simulink model "tank_PI"  (R2021a)
settings: Solver=FixedStepAuto  StartTime=0.0  StopTime=inf  FixedStep=0.1  RelTol=1e-3
model workspace (MATLAB code in the model file):
  | A1 = 1;
  | a1 = 0.1*0.1;
  | A2 = A1;
  | a2 = a1;
  | h10 = 1;
  | h20=1;
settings Model: EnablePacing=on  PacingRate=10  Creator=kjartan  LastModifiedBy=kjartan
settings SolverCC: AlgebraicLoopSolver=TrustRegion
settings DataIOCC: ReturnWorkspaceOutputs=off
settings DebuggingCC: SFMachineParentedDataDiag=warning  ArithmeticOperatorsInVariantConditions=warning
settings SFSimCC: CustomCodeUndefinedFunction=UseInterfaceOnly

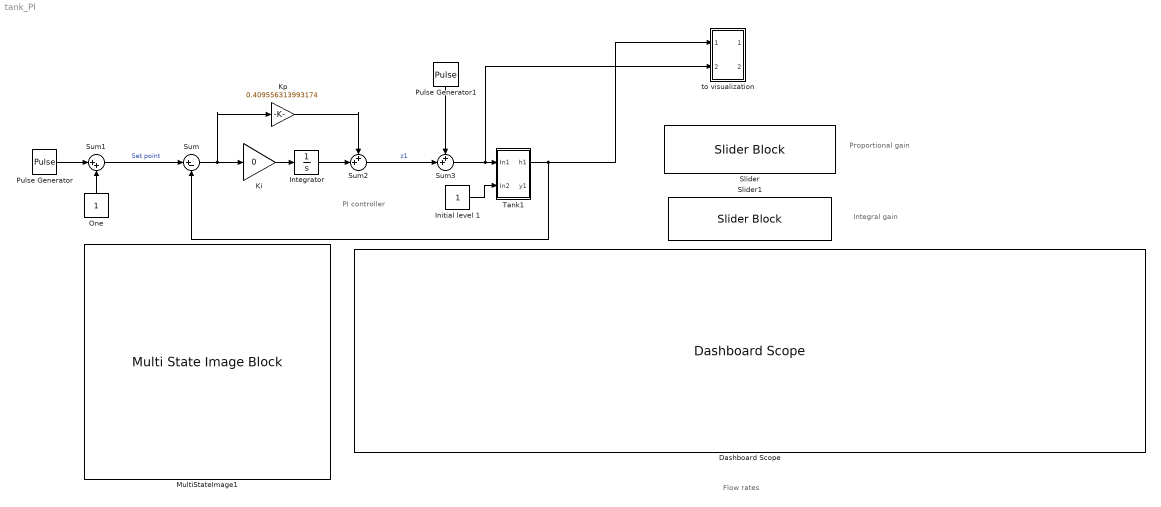
== system tank_PI ==
  note: Proportional gain
  note: Flow rates
  note: PI controller
  note: Integral gain
  Dashboard Scope : DashboardScope  Ymin=0  Ymax=2.5  ScaleAtStop=off
  Initial level 1 : Constant
  Integrator : Integrator
  Ki : Gain  Gain=0
  Kp : Gain  Gain=0.409556313993174
  MultiStateImage1 : MultiStateImageBlock
  One : Constant  OutDataTypeStr=Inherit: Inherit via back propagation
  Pulse Generator : DiscretePulseGenerator  PulseType=Time based  Amplitude=0.5  Period=60  PulseWidth=50
  Pulse Generator1 : DiscretePulseGenerator  PulseType=Time based  Amplitude=0.1  Period=60  PulseWidth=25  PhaseDelay=15
  Slider : SliderBlock  ScaleMax=2
  Slider1 : SliderBlock  ScaleMax=2
  Sum : Sum  Inputs=|+-
  Sum1 : Sum  Inputs=|++
  Sum2 : Sum  Inputs=++|
  Sum3 : Sum  Inputs=++|
  Tank1 : Subsystem
  to visualization : Subsystem
  wires:
  Tank1/1(h1) -> to visualization/1(In2), Sum/2
  Pulse Generator/1 -> Sum1/1
  Integrator/1 -> Sum2/2
  Sum/1 -> Kp/1, Ki/1
  Ki/1 -> Integrator/1
  Sum2/1 -> Sum3/2  "z1"
  Initial level 1/1 -> Tank1/2(In2)
  Kp/1 -> Sum2/1
  One/1 -> Sum1/2
  Sum1/1 -> Sum/1  "Set point"
  Sum3/1 -> to visualization/2(In3), Tank1/1(In1)
  Pulse Generator1/1 -> Sum3/1

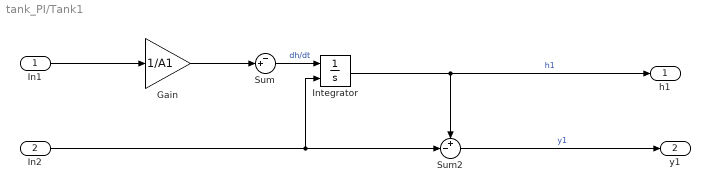
== system tank_PI/Tank1 ==
  In1 : Inport
  In2 : Inport  Port=2
  Gain : Gain  Gain=1/A1
  Integrator : Integrator  InitialConditionSource=external  InitialCondition=h10  LimitOutput=on  LowerSaturationLimit=0
  Sum : Sum  Inputs=-+|
  Sum2 : Sum  Inputs=+-|
  h1 : Outport  VectorParamsAs1DForOutWhenUnconnected=off
  y1 : Outport  Port=2  VectorParamsAs1DForOutWhenUnconnected=off
  wires:
  Gain/1 -> Sum/2
  Sum/1 -> Integrator/1  "dh/dt"
  In1/1 -> Gain/1
  Sum2/1 -> y1/1  "y1"
  Integrator/1 -> h1/1, Sum2/1  "h1"
  In2/1 -> Sum2/2, Integrator/2

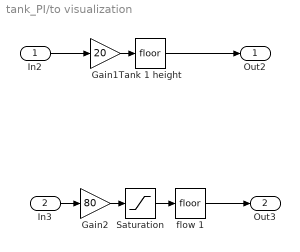
== system tank_PI/to visualization ==
  In2 : Inport
  In3 : Inport  Port=2
  Gain1 : Gain  Gain=20
  Gain2 : Gain  Gain=80
  Saturation : Saturate  UpperLimit=10  LowerLimit=0
  Tank 1 height : Rounding
  flow 1 : Rounding
  Out2 : Outport  VectorParamsAs1DForOutWhenUnconnected=off
  Out3 : Outport  Port=2  VectorParamsAs1DForOutWhenUnconnected=off
  wires:
  Tank 1 height/1 -> Out2/1
  Gain1/1 -> Tank 1 height/1
  In2/1 -> Gain1/1
  flow 1/1 -> Out3/1
  Gain2/1 -> Saturation/1
  In3/1 -> Gain2/1
  Saturation/1 -> flow 1/1
